simulink model "help_check"  (R2024b)
settings: Solver=FixedStepAuto  StartTime=0.0  StopTime=10.0  RelTol=1e-3
settings Model: Creator=makannan  LastModifiedBy=makannan

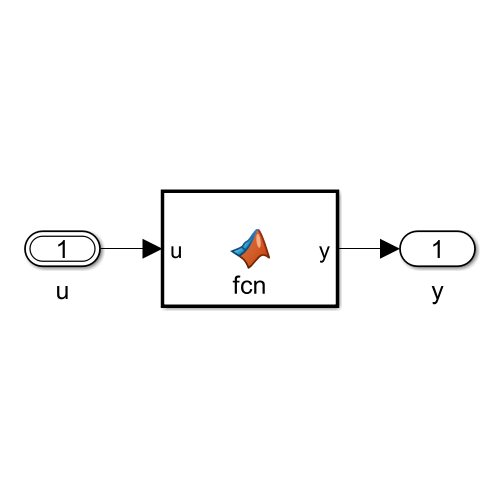
[thumbnail: Simulink's stored preview of the top-level diagram]
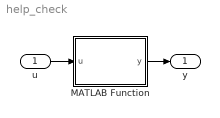
== system help_check ==
  u : Inport  OutDataTypeStr=Bus: GoalCheckInputBus
  MATLAB Function : MATLAB Function  TreatAsAtomicUnit=on
  y : Outport  OutDataTypeStr=double
  wires:
  u/1 -> MATLAB Function/1(u)
  MATLAB Function/1(y) -> y/1

== matlab function help_check/MATLAB Function ==
  data: u input Bus: GoalCheckInputBus; y output double
function y = fcn(u)

y = u.current_state.x;
